simulink model "Subsystem3"  (R2020a)
settings: Solver=VariableStepAuto  StartTime=0.0  StopTime=10.0  RelTol=1e-3
settings Model: Creator=anjal  LastModifiedBy=anjal
settings DataIOCC: SaveOutput=off  SaveTime=off

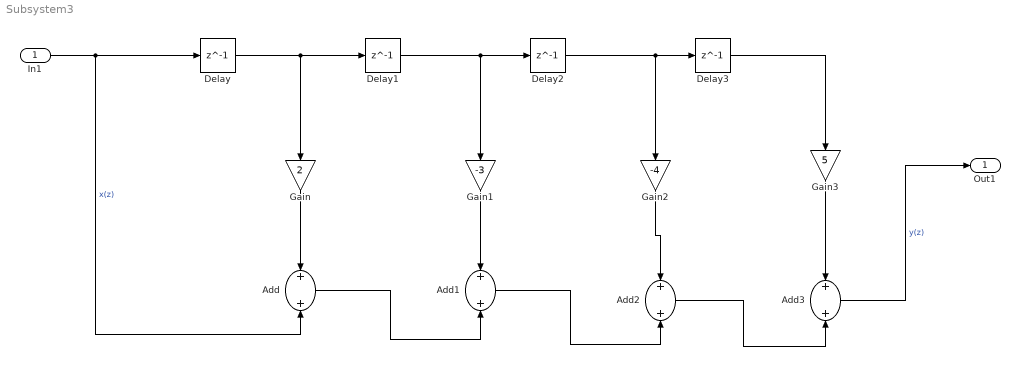
== system Subsystem3 ==
  In1 : Inport  OutDataTypeStr=double  PortDimensions=1  SampleTime=[0,1]
  Add{,1..3} (4 alike) : Sum
  Delay{,1..3} (4 alike) : Delay  DelayLength=1  InitialCondition=0
  Gain : Gain  Gain=2
  Gain1 : Gain  Gain=-3
  Gain2 : Gain  Gain=-4
  Gain3 : Gain  Gain=5
  Out1 : Outport  OutDataTypeStr=double  PortDimensions=1  SampleTime=[0,1]
  wires:
  Add1/1 -> Add2/2
  Delay1/1 -> Delay2/1, Gain1/1
  In1/1 -> Delay/1, Add/2  "x(z)"
  Add/1 -> Add1/2
  Add2/1 -> Add3/2
  Delay2/1 -> Delay3/1, Gain2/1
  Gain1/1 -> Add1/1
  Gain3/1 -> Add3/1
  Gain/1 -> Add/1
  Delay3/1 -> Gain3/1
  Delay/1 -> Delay1/1, Gain/1
  Gain2/1 -> Add2/1
  Add3/1 -> Out1/1  "y(z)"
